simulink model "PD"  (R2023b)
settings: Solver=VariableStepAuto  StartTime=0.0  StopTime=TF  RelTol=1e-3
undefined symbols (not defined in the file or in its folder): Obstacle, Target, x0
libraries: simulink x1
settings Model: Creator=isaiahthompson  LastModifiedBy=isaiahthompson

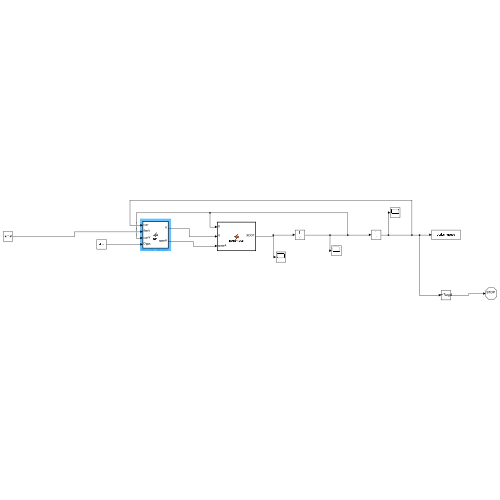
[thumbnail: Simulink's stored preview of the top-level diagram]
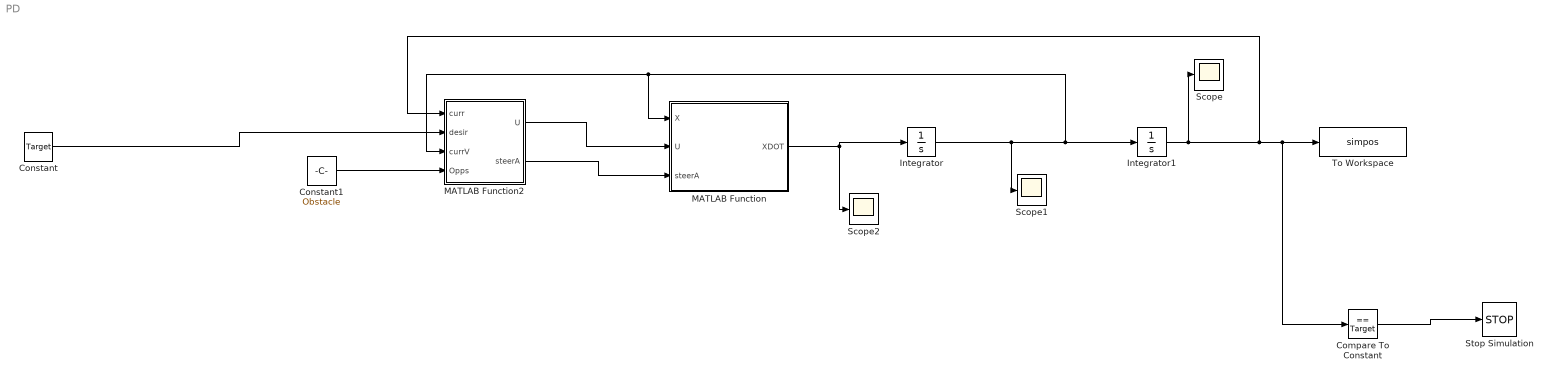
== system PD ==
  Compare To Constant : simulink/Logic and Bit Operations/Compare To Constant  relop===  const=Target  OutDataTypeStr=boolean
  Constant : Constant  Value=Target
  Constant1 : Constant  Value=Obstacle
  Integrator : Integrator  InitialCondition=x0
  Integrator1 : Integrator  InitialCondition=[0; 0]
  MATLAB Function : MATLAB Function  TreatAsAtomicUnit=on
  MATLAB Function2 : MATLAB Function  TreatAsAtomicUnit=on
  Scope : Scope
  Scope1 : Scope
  Scope2 : Scope
  Stop Simulation : Stop
  To Workspace : ToWorkspace  VariableName=simpos  SaveFormat=Structure With Time  SampleTime=-1
  wires:
  MATLAB Function/1(XDOT) -> Integrator/1, Scope2/1
  Integrator/1 -> Scope1/1, MATLAB Function/1(X), MATLAB Function2/3(currV), Integrator1/1
  Integrator1/1 -> Scope/1, To Workspace/1, Compare To Constant/1, MATLAB Function2/1(curr)
  Constant/1 -> MATLAB Function2/2(desir)
  MATLAB Function2/1(U) -> MATLAB Function/2(U)
  Compare To Constant/1 -> Stop Simulation/1
  Constant1/1 -> MATLAB Function2/4(Opps)
  MATLAB Function2/2(steerA) -> MATLAB Function/3(steerA)

== matlab function PD/MATLAB Function ==
  data: X input; XDOT output; U input; steerA input
function XDOT    = pointmass(X,U,steerA)

m = 3
g = 9.81

%State Variables
x1 = X(1) %U
x2 = X(2) %V

%Control Variables

% U(1) = m * g * u3 * sin(o)
% U(2) = m * g * u3 * cos(o)

u1 = U(1) * m %Forces x
u2 = U(2) * m %Forces y
%u3 = U(3) %throttle position
IntAng = atand(u1/u2)

%Determine the direction of vehicle's velocity
o = atand(x1/x2)
b = 30
%Speed of V
Va = sqrt(x1^2 + x2^2)


%Forces

%Engine
Fengx = m * g * sind(o)
Fengy = m * g *  cosd(o)
Feng = sqrt(Fengx^2 + Fengy^2)

%Drag
Fdragx = -0.35 * Va^2 * sind(o)
Fdragy = -0.35 * Va^2 * cosd(o)
Fdrag = sqrt(Fdragx^2 + Fdragy^2)

%Wind
Fwx = 30*sind(b) % Model Wave as a sine wave
Fwy = 30*cosd(b)

w_o = b
if w_o >= 0 & w_o <= 90
    Fwx = Fwx
    Fwy = Fwy
elseif w_o >= 90 & w_o <= 180
    Fwx = Fwx
    Fwy = -Fwy
elseif w_o >= 180 & w_o <= 270
    Fwx = -Fwx
    Fwy = -Fwy
else
    Fwx = -Fwx
    Fwy = Fwy
end
Fw = sqrt(Fwx^2 + Fwy^2)
% navX = steerA(1) * m
% navY = steerA(2) * m
Fx = Fengx + Fdragx + Fwx + u1 
Fy = Fengy + Fdragy + Fwy + u2 

%Acceleration
ax = (Fx/m) 
ay = (Fy/m) 
a = sqrt(ax^2 + ay^2)
A = [ax;
     ay];

dotP = dot(U,A)
errorAng = acosd(complex(dotP))

errorA = U - A
% PropK = 7
% errorVV = PropK * errorV

XDOT = [ax;ay]

end

== matlab function PD/MATLAB Function2 ==
  data: curr input; U output; desir input; currV input; Opps input; steerA output
function [U,steerA]  = fcn(curr,desir,currV,Opps)
error = desir - curr
numOpps = length(Opps(1,:))
% for x = 1:numOpps
%     diff = abs(Opps(x,:) - curr)
%     if diff(1) <= 25 & diff(2) <= 25
%         oppsAV = 1
%         steerAx = -diff(1) * 30
%         steerAy = -diff(2) * 30
%     % elseif diff(1) <= 25 & diff(2) > 25
%     %     oppsAV = 1
%     %     steerAx = -diff(1) * 30
%     %     steerAy = 0
%     % elseif diff(1) > 25 & diff(2) <= 25
%     %     oppsAV = 1
%     %     steerAx = 0
%     %     steerAy = -diff(2) * 30
%     else
%         oppsAV = 0
%         steerAx = 0
%         steerAy = 0
%     end
% end 

Kp = 2
Kd = 3
if oppsAV == 1
    Kp = 0
    Kd = 0
else
    Kp = Kp
    Kd = Kd
end

%ax = Kp * error(1) - Kd * currV(1) + steerAx
%ay = Kp * error(2) - Kd * currV(2) + steerAy

ax = Kp * error(1) - Kd * currV(1) 
ay = Kp * error(2) - Kd * currV(2) 

U = [ax;
     ay];
steerA = [steerAx;
          steerAy];
